simulink model "Cell_ModelSim"  (R2021a)
settings: Solver=VariableStepAuto  StartTime=0.0  StopTime=sim_time  RelTol=1e-3
values from neighbouring files (symbols this model uses):
  Cn = (2*3600)    (= 7200)    [Cell_Model.m]
  i = 2    [Cell_Model.m]
  ocv = data(:,2)    [Cell_Model.m]
  r_discharge = data(:,4)    [Cell_Model.m]
  soc = data(:,1)    [Cell_Model.m]
settings Model: Creator=Samiran  LastModifiedBy=Samiran

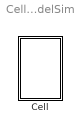
== system Cell_ModelSim ==
  Cell : Subsystem

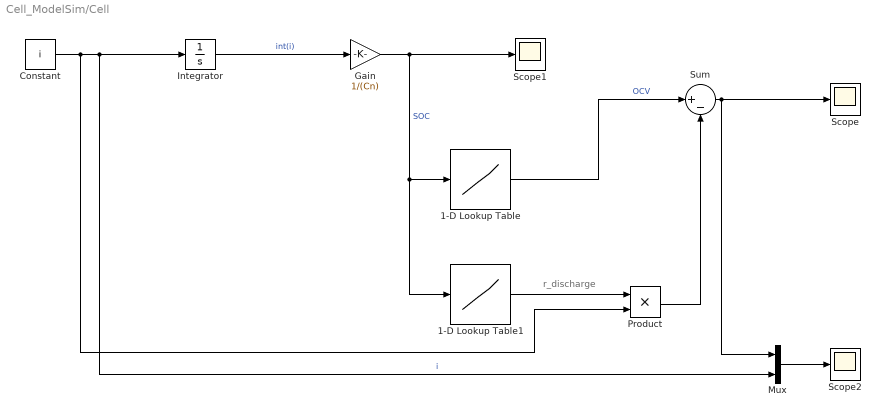
== system Cell_ModelSim/Cell ==
  note: r_discharge
  1-D Lookup Table : Lookup_n-D  NumberOfTableDimensions=1  BreakpointsForDimension1=soc  Table=ocv  InternalRulePriority=Speed  RndMeth=Simplest  InputSameDT=on
  1-D Lookup Table1 : Lookup_n-D  NumberOfTableDimensions=1  BreakpointsForDimension1=soc  Table=r_discharge  InternalRulePriority=Speed  RndMeth=Simplest  InputSameDT=on
  Constant : Constant  Value=i
  Gain : Gain  Gain=1/(Cn)
  Integrator : Integrator
  Mux : Mux  Inputs=2
  Product : Product
  Scope : Scope
  Scope1 : Scope
  Scope2 : Scope
  Sum : Sum  Inputs=|+-
  wires:
  1-D Lookup Table/1 -> Sum/1  "OCV"
  Mux/1 -> Scope2/1
  Sum/1 -> Mux/1, Scope/1
  Product/1 -> Sum/2
  1-D Lookup Table1/1 -> Product/1
  Integrator/1 -> Gain/1  "int(i)"
  Gain/1 -> Scope1/1, 1-D Lookup Table1/1, 1-D Lookup Table/1  "SOC"
  Constant/1 -> Product/2, Mux/2, Integrator/1  "i"
